simulink subsystem "local_control_example"  (R2022b)
settings: Solver=VariableStepAuto  StartTime=0.0  StopTime=10.0  RelTol=1e-3
undefined symbols (not defined in the file): route1_waypoint_raw
libraries: CarMaker4SL x7
settings Model: Creator=USER  LastModifiedBy=USER

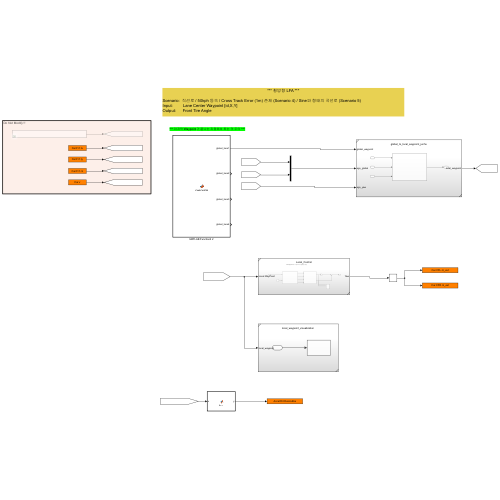
[thumbnail: Simulink's stored preview of the top-level diagram]
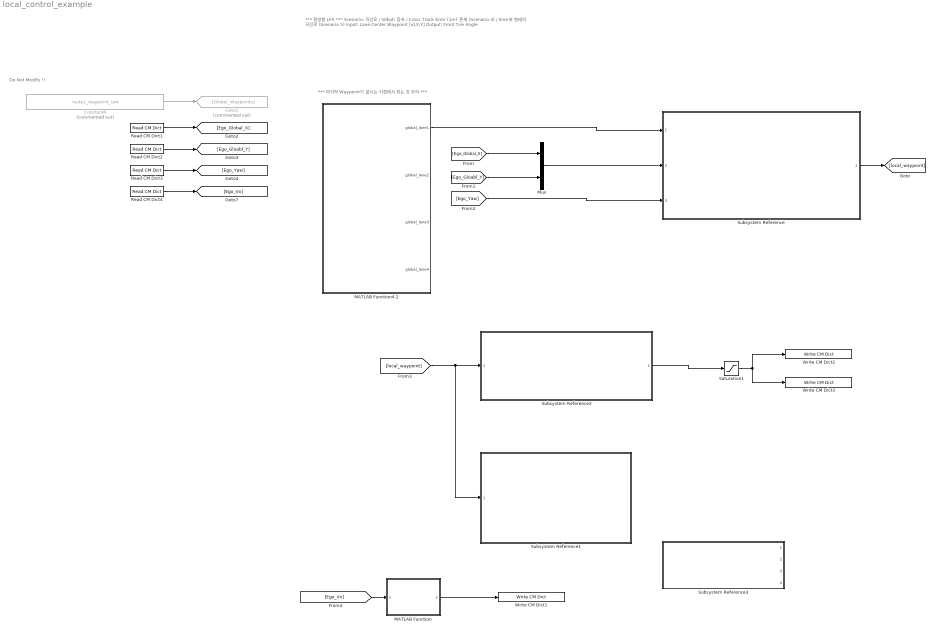
== system local_control_example ==
  note: *** 횡방향 LFA ***
      |
      | Scenario: 직선로 / 50kph 등속 / Cross Track Error (1m) 존재 (Scenario 4) / Sine파 형태의 곡선로 (Scenario 5)
      | Input: Lane Center Waypoint [id,X,Y]
      | Output: Front Tire Angle
  note: *** 마지막 Waypoint가 끝나는 지점에서 튀는 것 주의 ***
  note: Do Not Modify !!
  Constant4 : Constant  Commented=on  Value=route1_waypoint_raw
  Goto1 : Goto  Commented=on  GotoTag=Global_Waypoints
  MATLAB Function : MATLAB Function  TreatAsAtomicUnit=on
  MATLAB Function4 2 : MATLAB Function  TreatAsAtomicUnit=on
  Mux : Mux  Inputs=2
  Read CM Dict1 : CarMaker4SL/Read CM Dict  xname=Car.Fr1.tx  xsync=off  xstime=Inherited
  Read CM Dict2 : CarMaker4SL/Read CM Dict  xname=Car.Fr1.ty  xsync=off  xstime=Inherited
  Read CM Dict3 : CarMaker4SL/Read CM Dict  xname=Car.Fr1.rz  xsync=off  xstime=Inherited
  Read CM Dict4 : CarMaker4SL/Read CM Dict  xname=Car.v  xsync=off  xstime=Inherited
  Saturation1 : Saturate  UpperLimit=2  LowerLimit=-2
  Subsystem Reference : Subsystem  ReferencedSubsystem=global_to_local_waypoint_junho
  Subsystem Reference1 : Subsystem  ReferencedSubsystem=local_waypoint_visualization
  Subsystem Reference2 : Subsystem  ReferencedSubsystem=Local_Control
  Subsystem Reference3 : Subsystem  ReferencedSubsystem=Get_Traffic_by_Line
  Write CM Dict1 : CarMaker4SL/Write CM Dict  xname=AccelCtrl.DesiredAx  xsync=off
  Write CM Dict2 : CarMaker4SL/Write CM Dict  xname=Car.CFL.rz_ext  xsync=off
  Write CM Dict3 : CarMaker4SL/Write CM Dict  xname=Car.CFR.rz_ext  xsync=off
  wires:
  MATLAB Function/1(y) -> Write CM Dict1/1
  Constant4/1 -> Goto1/1
  [Ego_Vx] -> MATLAB Function/1(u)
  Subsystem Reference/1 -> [local_waypoint]
  [local_waypoint] -> Subsystem Reference2/1, Subsystem Reference1/1
  Read CM Dict2/1 -> [Ego_Gloabl_Y]
  MATLAB Function4 2/1(global_lane1) -> Subsystem Reference/1
  Subsystem Reference2/1 -> Saturation1/1
  [Ego_Gloabl_Y] -> Mux/2
  Saturation1/1 -> Write CM Dict2/1, Write CM Dict3/1
  Mux/1 -> Subsystem Reference/2
  Read CM Dict1/1 -> [Ego_Global_X]
  [Ego_Global_X] -> Mux/1
  Read CM Dict4/1 -> [Ego_Vx]
  [Ego_Yaw] -> Subsystem Reference/3
  Read CM Dict3/1 -> [Ego_Yaw]

== matlab function local_control_example/MATLAB Function4 2 ==
  settings: sampleTime=0.1
  data: global_lane1 output; global_lane2 output; global_lane3 output; global_lane4 output
function [global_lane1, global_lane2, global_lane3, global_lane4] = CHECKER()

    %% Localization plotter
    f1 = load('Song_waypoints_data.mat');
    f2 = load('Song_roadprofiles_data.mat');

    n_waypoint = height(f1.ids);
    n_roadprofile = height(f2.ids);

    % 미리 고정된 크기의 큰 배열로 초기화
    max_size = 1000; % 필요에 따라 적절한 값으로 설정
    global_lane1 = NaN(max_size, 2); % NaN으로 초기화하여 미리 고정 크기를 설정
    global_lane2 = NaN(max_size, 2);
    global_lane3 = NaN(max_size, 2);
    global_lane4 = NaN(max_size, 2);

    lane1_idx = 1;
    lane2_idx = 1;
    lane3_idx = 1;
    lane4_idx = 1;

    % Loop through each road profile
    for i = 1 : n_roadprofile
        x = zeros(1, 50);
        y = zeros(1, 50);
        idx = 1;

        for j = 1:50
            if f2.waypoints(i,j) ~= 0
                x(idx) = f1.waypoints(f2.waypoints(i,j),1);
                y(idx) = f1.waypoints(f2.waypoints(i,j),2);

                if x(idx) >= -200 && x(idx) <= 200 && y(idx) >= -200 && y(idx) <= 200
                    idx = idx + 1;
                end
            end
        end

        % 유효한 값을 각 lane에 추가
        if ismember(i, 1:10)
            global_lane1(lane1_idx:lane1_idx+idx-2, :) = [x(1:idx-1)', y(1:idx-1)'];
            lane1_idx = lane1_idx + idx - 1;
        elseif ismember(i, 11:20)
            global_lane2(lane2_idx:lane2_idx+idx-2, :) = [x(1:idx-1)', y(1:idx-1)'];
            lane2_idx = lane2_idx + idx - 1;
        elseif ismember(i, 21:30)
            global_lane3(lane3_idx:lane3_idx+idx-2, :) = [x(1:idx-1)', y(1:idx-1)'];
            lane3_idx = lane3_idx + idx - 1;
        elseif ismember(i, 31:33)
            global_lane4(lane4_idx:lane4_idx+idx-2, :) = [x(1:idx-1)', y(1:idx-1)'];
            lane4_idx = lane4_idx + idx - 1;
        end
    end

    % 더 이상 할당할 필요 없이 global_lane을 그대로 사용
end

== matlab function local_control_example/MATLAB Function ==
  data: u input; y output
function y = fcn(u)
    y =  0;
    if u * 3.8 < 50
        y = 1;
    else
        y = -1;
    end 
end
